simulink model "chap5_11sim"  (Simulink 5.0)
settings: Solver=ode45  StartTime=0.0  StopTime=20  RelTol=1e-3
settings Model: LastModifiedBy=Administrator  ExtModeTrigMode=oneshot  ExtModeArmWhenConnect=off  SaveTime=off  SaveOutput=off  Decimation=100  LimitDataPoints=off  BooleanDataType=off

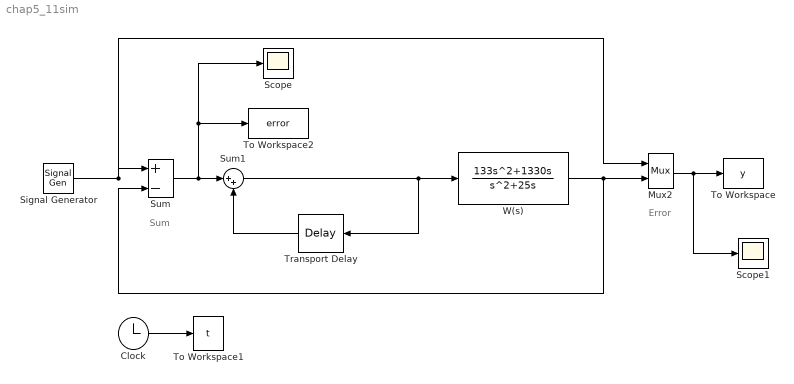
== system chap5_11sim ==
  note: Sum
  note: Error
  Clock : Clock
      settings: Decimation=10
  Mux2 : Mux  Inputs=2
  Scope : Scope
      settings: TimeRange=1  YMin=-0.0001  YMax=0.00055  MaxDataPoints=500000  Decimation=0.001  SampleInput=on  SampleTime=0.001
  Scope1 : Scope
      settings: TimeRange=1  YMin=-0.0001  YMax=0.00055  MaxDataPoints=500000  Decimation=0.001  SampleInput=on  SampleTime=0.001
  Signal Generator : SignalGenerator  Amplitude=0.5  Frequency=0.5
  Sum : Sum  Inputs=|+-  SaturateOnIntegerOverflow=on  InputSameDT=on
  Sum1 : Sum  Inputs=|++  SaturateOnIntegerOverflow=on  InputSameDT=on
  To Workspace : ToWorkspace  VariableName=y  SampleTime=-1  SaveFormat=Array
  To Workspace1 : ToWorkspace  VariableName=t  SampleTime=-1  SaveFormat=Array
  To Workspace2 : ToWorkspace  VariableName=error  SampleTime=-1  SaveFormat=Array
  Transport Delay : TransportDelay  Orientation=left  DelayTime=2  BufferSize=10240  TransDelayFeedthrough=on
  W(s) : TransferFcn  Numerator=[133 1330 0]  Denominator=[1 25 0]
  wires:
  Mux2/1 -> To Workspace/1, Scope1/1
  Sum/1 -> Sum1/1, Scope/1, To Workspace2/1
  Signal Generator/1 -> Sum/1, Mux2/1
  Sum1/1 -> Transport Delay/1, W(s)/1
  Transport Delay/1 -> Sum1/2
  W(s)/1 -> Mux2/2, Sum/2
  Clock/1 -> To Workspace1/1
